simulink model "AcO_Ctrl_Geometric_headless_R2016a"  (R2016a)
settings: Solver=FixedStepDiscrete  StartTime=0.0  StopTime=simulation_duration  FixedStep=Ts  RelTol=1e-3
values from neighbouring files (symbols this model uses):
  M1_BeMo_d = zeros(7,M1_n_mode)    [AcO_Ctrl_headless_cfg.m]    (also in agws_cfg.m = 1e-6*bsxfun(@times,randn(7,M1_n_mode),scale); agws_fastTT_cfg.m = 1e-6*bsxfun(@times,randn(7,M1_n_mode),scale))
  M1_RiBo_d = zeros(7,6)    [AcO_Ctrl_headless_cfg.m]    (also in agws_cfg.m = [M1_Txyz0 M1_Rxyz0]; agws_fastTT_cfg.m = [M1_Txyz0 M1_Rxyz0])
  M2_RiBo_d = zeros(7,6)    [AcO_Ctrl_headless_cfg.m]    (also in agws_cfg.m = [M2_Txyz0 M2_Rxyz0]; agws_fastTT_cfg.m = [M2_Txyz0 M2_Rxyz0])
  Ts = 1/fs    (= 0.002)    [AcO_Ctrl_headless_cfg.m]    (also in agws_fastTT_cfg.m = 0.005)
undefined symbols (not defined in the file or in its folder): Az_C, CG2Hp, CG2Hp_S7, El_C, Fsmm, GIR_C, Hp2CG_f, Hp2CG_f_S7, HPdtf, HpK, KM2, M2_actdyn, M2_CG2Hp, M_LOS, MIMO_C, PTT2act, PTT2act_even, Q, sysd, TT2act, TT2act_even
undefined symbols (not defined in the file): on_axis_src_outputs
libraries: CEO x2
(part 5 of 6)

== system AcO_Ctrl_Geometric_headless_R2016a/Structural Dynamics V3.3/Structural Dynamics V3.3a/Structural Dynamics Plus CL Az El M1 force/M1 Sensing/senseM1S2 ==
  HP_D_cmd : Inport
  HP_D_face : Inport  Port=2
  HP_D_cell : Inport  Port=3
  Hp2CG_f : Gain  Gain=Hp2CG_f  Multiplication=Matrix(K*u)
  KHp : Gain  Gain=-HpK
  Sum1 : Sum  Inputs=-+|
  Sum9 : Sum  Inputs=-+|
  HardPoint_6DOF_Force : Outport
  wires:
  HP_D_face/1 -> Sum9/2
  HP_D_cmd/1 -> Sum1/1
  HP_D_cell/1 -> Sum9/1
  Hp2CG_f/1 -> HardPoint_6DOF_Force/1
  Sum9/1 -> Sum1/2
  Sum1/1 -> KHp/1
  KHp/1 -> Hp2CG_f/1

== system AcO_Ctrl_Geometric_headless_R2016a/Structural Dynamics V3.3/Structural Dynamics V3.3a/Structural Dynamics Plus CL Az El M1 force/M1 Sensing/senseM1S3 ==
  HP_D_cmd : Inport
  HP_D_face : Inport  Port=2
  HP_D_cell : Inport  Port=3
  Hp2CG_f : Gain  Gain=Hp2CG_f  Multiplication=Matrix(K*u)
  KHp : Gain  Gain=-HpK
  Sum1 : Sum  Inputs=-+|
  Sum9 : Sum  Inputs=-+|
  HardPoint_6DOF_Force : Outport
  wires:
  Hp2CG_f/1 -> HardPoint_6DOF_Force/1
  HP_D_cell/1 -> Sum9/1
  HP_D_cmd/1 -> Sum1/1
  HP_D_face/1 -> Sum9/2
  Sum9/1 -> Sum1/2
  Sum1/1 -> KHp/1
  KHp/1 -> Hp2CG_f/1

== system AcO_Ctrl_Geometric_headless_R2016a/Structural Dynamics V3.3/Structural Dynamics V3.3a/Structural Dynamics Plus CL Az El M1 force/M1 Sensing/senseM1S4 ==
  HP_D_cmd : Inport
  HP_D_face : Inport  Port=2
  HP_D_cell : Inport  Port=3
  Hp2CG_f : Gain  Gain=Hp2CG_f  Multiplication=Matrix(K*u)
  KHp : Gain  Gain=-HpK
  Sum1 : Sum  Inputs=-+|
  Sum9 : Sum  Inputs=-+|
  HardPoint_6DOF_Force : Outport
  wires:
  HP_D_face/1 -> Sum9/2
  HP_D_cmd/1 -> Sum1/1
  HP_D_cell/1 -> Sum9/1
  Hp2CG_f/1 -> HardPoint_6DOF_Force/1
  Sum9/1 -> Sum1/2
  Sum1/1 -> KHp/1
  KHp/1 -> Hp2CG_f/1

== system AcO_Ctrl_Geometric_headless_R2016a/Structural Dynamics V3.3/Structural Dynamics V3.3a/Structural Dynamics Plus CL Az El M1 force/M1 Sensing/senseM1S5 ==
  HP_D_cmd : Inport
  HP_D_face : Inport  Port=2
  HP_D_cell : Inport  Port=3
  Hp2CG_f : Gain  Gain=Hp2CG_f  Multiplication=Matrix(K*u)
  KHp : Gain  Gain=-HpK
  Sum1 : Sum  Inputs=-+|
  Sum9 : Sum  Inputs=-+|
  HardPoint_6DOF_Force : Outport
  wires:
  Hp2CG_f/1 -> HardPoint_6DOF_Force/1
  HP_D_cell/1 -> Sum9/1
  HP_D_cmd/1 -> Sum1/1
  HP_D_face/1 -> Sum9/2
  Sum9/1 -> Sum1/2
  Sum1/1 -> KHp/1
  KHp/1 -> Hp2CG_f/1

== system AcO_Ctrl_Geometric_headless_R2016a/Structural Dynamics V3.3/Structural Dynamics V3.3a/Structural Dynamics Plus CL Az El M1 force/M1 Sensing/senseM1S6 ==
  HP_D_cmd : Inport
  HP_D_face : Inport  Port=2
  HP_D_cell : Inport  Port=3
  Hp2CG_f : Gain  Gain=Hp2CG_f  Multiplication=Matrix(K*u)
  KHp : Gain  Gain=-HpK
  Sum1 : Sum  Inputs=-+|
  Sum9 : Sum  Inputs=-+|
  HardPoint_6DOF_Force : Outport
  wires:
  HP_D_face/1 -> Sum9/2
  HP_D_cmd/1 -> Sum1/1
  HP_D_cell/1 -> Sum9/1
  Hp2CG_f/1 -> HardPoint_6DOF_Force/1
  Sum9/1 -> Sum1/2
  Sum1/1 -> KHp/1
  KHp/1 -> Hp2CG_f/1

== system AcO_Ctrl_Geometric_headless_R2016a/Structural Dynamics V3.3/Structural Dynamics V3.3a/Structural Dynamics Plus CL Az El M1 force/M1 Sensing/senseM1S7 ==
  HP_D_cmd : Inport
  HP_D_face : Inport  Port=2
  HP_D_cell : Inport  Port=3
  Hp2CG_f_S7 : Gain  Gain=Hp2CG_f_S7  Multiplication=Matrix(K*u)
  KHp : Gain  Gain=-HpK
  Sum1 : Sum  Inputs=-+|
  Sum9 : Sum  Inputs=-+|
  HardPoint_6DOF_Force : Outport
  wires:
  Hp2CG_f_S7/1 -> HardPoint_6DOF_Force/1
  HP_D_cell/1 -> Sum9/1
  HP_D_cmd/1 -> Sum1/1
  HP_D_face/1 -> Sum9/2
  Sum9/1 -> Sum1/2
  Sum1/1 -> KHp/1
  KHp/1 -> Hp2CG_f_S7/1

== system AcO_Ctrl_Geometric_headless_R2016a/Structural Dynamics V3.3/Structural Dynamics V3.5.2/Structural Dynamics Plus CL Az El M1 force/M1 Force Control/ControlM1S1 ==
  In1 : Inport
  -1(2)3 : Gain  Gain=-1
  Actuator Model : DiscreteStateSpace  A=Q.A  B=Q.B  C=Q.C  D=Q.D  SampleTime=1/Fsmm
  MIMO Controller : Subsystem
  Out1 : Outport
  Out2 : Outport  Port=2
  wires:
  MIMO Controller/1(Out1) -> Actuator Model/1
  -1(2)3/1 -> Out2/1
  Actuator Model/1 -> -1(2)3/1, Out1/1
  In1/1 -> MIMO Controller/1(In1)

== system AcO_Ctrl_Geometric_headless_R2016a/Structural Dynamics V3.3/Structural Dynamics V3.5.2/Structural Dynamics Plus CL Az El M1 force/M1 Force Control/ControlM1S2 ==
  In1 : Inport
  -1(2)3 : Gain  Gain=-1
  Actuator Model : DiscreteStateSpace  A=Q.A  B=Q.B  C=Q.C  D=Q.D  SampleTime=1/Fsmm
  MIMO Controller : Subsystem
  Out1 : Outport
  Out2 : Outport  Port=2
  wires:
  In1/1 -> MIMO Controller/1(In1)
  Actuator Model/1 -> Out1/1, -1(2)3/1
  -1(2)3/1 -> Out2/1
  MIMO Controller/1(Out1) -> Actuator Model/1

== system AcO_Ctrl_Geometric_headless_R2016a/Structural Dynamics V3.3/Structural Dynamics V3.5.2/Structural Dynamics Plus CL Az El M1 force/M1 Force Control/ControlM1S3 ==
  In1 : Inport
  -1(2)3 : Gain  Gain=-1
  Actuator Model : DiscreteStateSpace  A=Q.A  B=Q.B  C=Q.C  D=Q.D  SampleTime=1/Fsmm
  MIMO Controller : Subsystem
  Out1 : Outport
  Out2 : Outport  Port=2
  wires:
  MIMO Controller/1(Out1) -> Actuator Model/1
  -1(2)3/1 -> Out2/1
  Actuator Model/1 -> -1(2)3/1, Out1/1
  In1/1 -> MIMO Controller/1(In1)

== system AcO_Ctrl_Geometric_headless_R2016a/Structural Dynamics V3.3/Structural Dynamics V3.5.2/Structural Dynamics Plus CL Az El M1 force/M1 Force Control/ControlM1S4 ==
  In1 : Inport
  -1(2)3 : Gain  Gain=-1
  Actuator Model : DiscreteStateSpace  A=Q.A  B=Q.B  C=Q.C  D=Q.D  SampleTime=1/Fsmm
  MIMO Controller : Subsystem
  Out1 : Outport
  Out2 : Outport  Port=2
  wires:
  In1/1 -> MIMO Controller/1(In1)
  Actuator Model/1 -> Out1/1, -1(2)3/1
  -1(2)3/1 -> Out2/1
  MIMO Controller/1(Out1) -> Actuator Model/1

== system AcO_Ctrl_Geometric_headless_R2016a/Structural Dynamics V3.3/Structural Dynamics V3.5.2/Structural Dynamics Plus CL Az El M1 force/M1 Force Control/ControlM1S5 ==
  In1 : Inport
  -1(2)3 : Gain  Gain=-1
  Actuator Model : DiscreteStateSpace  A=Q.A  B=Q.B  C=Q.C  D=Q.D  SampleTime=1/Fsmm
  MIMO Controller : Subsystem
  Out1 : Outport
  Out2 : Outport  Port=2
  wires:
  MIMO Controller/1(Out1) -> Actuator Model/1
  -1(2)3/1 -> Out2/1
  Actuator Model/1 -> -1(2)3/1, Out1/1
  In1/1 -> MIMO Controller/1(In1)

== system AcO_Ctrl_Geometric_headless_R2016a/Structural Dynamics V3.3/Structural Dynamics V3.5.2/Structural Dynamics Plus CL Az El M1 force/M1 Force Control/ControlM1S6 ==
  In1 : Inport
  -1(2)3 : Gain  Gain=-1
  Actuator Model : DiscreteStateSpace  A=Q.A  B=Q.B  C=Q.C  D=Q.D  SampleTime=1/Fsmm
  MIMO Controller : Subsystem
  Out1 : Outport
  Out2 : Outport  Port=2
  wires:
  In1/1 -> MIMO Controller/1(In1)
  Actuator Model/1 -> Out1/1, -1(2)3/1
  -1(2)3/1 -> Out2/1
  MIMO Controller/1(Out1) -> Actuator Model/1

== system AcO_Ctrl_Geometric_headless_R2016a/Structural Dynamics V3.3/Structural Dynamics V3.5.2/Structural Dynamics Plus CL Az El M1 force/M1 Force Control/ControlM1S7 ==
  In1 : Inport
  -1(2)3 : Gain  Gain=-1
  Actuator Model : DiscreteStateSpace  A=Q.A  B=Q.B  C=Q.C  D=Q.D  SampleTime=1/Fsmm
  MIMO Controller : Subsystem
  Out1 : Outport
  Out2 : Outport  Port=2
  wires:
  MIMO Controller/1(Out1) -> Actuator Model/1
  -1(2)3/1 -> Out2/1
  Actuator Model/1 -> -1(2)3/1, Out1/1
  In1/1 -> MIMO Controller/1(In1)

== system AcO_Ctrl_Geometric_headless_R2016a/Structural Dynamics V3.3/Structural Dynamics V3.5.2/Structural Dynamics Plus CL Az El M1 force/M1 Sensing/senseM1S1 ==
  HP_D_cmd : Inport
  HP_D_face : Inport  Port=2
  HP_D_cell : Inport  Port=3
  Hp2CG_f : Gain  Gain=Hp2CG_f  Multiplication=Matrix(K*u)
  KHp : Gain  Gain=-HpK
  Sum1 : Sum  Inputs=-+|
  Sum9 : Sum  Inputs=-+|
  HardPoint_6DOF_Force : Outport
  wires:
  Hp2CG_f/1 -> HardPoint_6DOF_Force/1
  HP_D_cell/1 -> Sum9/1
  HP_D_cmd/1 -> Sum1/1
  HP_D_face/1 -> Sum9/2
  Sum9/1 -> Sum1/2
  Sum1/1 -> KHp/1
  KHp/1 -> Hp2CG_f/1

== system AcO_Ctrl_Geometric_headless_R2016a/Structural Dynamics V3.3/Structural Dynamics V3.5.2/Structural Dynamics Plus CL Az El M1 force/M1 Sensing/senseM1S2 ==
  HP_D_cmd : Inport
  HP_D_face : Inport  Port=2
  HP_D_cell : Inport  Port=3
  Hp2CG_f : Gain  Gain=Hp2CG_f  Multiplication=Matrix(K*u)
  KHp : Gain  Gain=-HpK
  Scope : Scope
  Sum1 : Sum  Inputs=-+|
  Sum9 : Sum  Inputs=-+|
  HardPoint_6DOF_Force : Outport
  wires:
  HP_D_face/1 -> Sum9/2
  HP_D_cmd/1 -> Sum1/1
  Sum9/1 -> Scope/1, Sum1/2
  KHp/1 -> Hp2CG_f/1
  Hp2CG_f/1 -> HardPoint_6DOF_Force/1
  Sum1/1 -> KHp/1
  HP_D_cell/1 -> Sum9/1

== system AcO_Ctrl_Geometric_headless_R2016a/Structural Dynamics V3.3/Structural Dynamics V3.5.2/Structural Dynamics Plus CL Az El M1 force/M1 Sensing/senseM1S3 ==
  HP_D_cmd : Inport
  HP_D_face : Inport  Port=2
  HP_D_cell : Inport  Port=3
  Hp2CG_f : Gain  Gain=Hp2CG_f  Multiplication=Matrix(K*u)
  KHp : Gain  Gain=-HpK
  Sum1 : Sum  Inputs=-+|
  Sum9 : Sum  Inputs=-+|
  HardPoint_6DOF_Force : Outport
  wires:
  HP_D_face/1 -> Sum9/2
  HP_D_cmd/1 -> Sum1/1
  HP_D_cell/1 -> Sum9/1
  Hp2CG_f/1 -> HardPoint_6DOF_Force/1
  Sum9/1 -> Sum1/2
  Sum1/1 -> KHp/1
  KHp/1 -> Hp2CG_f/1

== system AcO_Ctrl_Geometric_headless_R2016a/Structural Dynamics V3.3/Structural Dynamics V3.5.2/Structural Dynamics Plus CL Az El M1 force/M1 Sensing/senseM1S4 ==
  HP_D_cmd : Inport
  HP_D_face : Inport  Port=2
  HP_D_cell : Inport  Port=3
  Hp2CG_f : Gain  Gain=Hp2CG_f  Multiplication=Matrix(K*u)
  KHp : Gain  Gain=-HpK
  Sum1 : Sum  Inputs=-+|
  Sum9 : Sum  Inputs=-+|
  HardPoint_6DOF_Force : Outport
  wires:
  Hp2CG_f/1 -> HardPoint_6DOF_Force/1
  HP_D_cell/1 -> Sum9/1
  HP_D_cmd/1 -> Sum1/1
  HP_D_face/1 -> Sum9/2
  Sum9/1 -> Sum1/2
  Sum1/1 -> KHp/1
  KHp/1 -> Hp2CG_f/1

== system AcO_Ctrl_Geometric_headless_R2016a/Structural Dynamics V3.3/Structural Dynamics V3.5.2/Structural Dynamics Plus CL Az El M1 force/M1 Sensing/senseM1S5 ==
  HP_D_cmd : Inport
  HP_D_face : Inport  Port=2
  HP_D_cell : Inport  Port=3
  Hp2CG_f : Gain  Gain=Hp2CG_f  Multiplication=Matrix(K*u)
  KHp : Gain  Gain=-HpK
  Sum1 : Sum  Inputs=-+|
  Sum9 : Sum  Inputs=-+|
  HardPoint_6DOF_Force : Outport
  wires:
  HP_D_face/1 -> Sum9/2
  HP_D_cmd/1 -> Sum1/1
  HP_D_cell/1 -> Sum9/1
  Hp2CG_f/1 -> HardPoint_6DOF_Force/1
  Sum9/1 -> Sum1/2
  Sum1/1 -> KHp/1
  KHp/1 -> Hp2CG_f/1

== system AcO_Ctrl_Geometric_headless_R2016a/Structural Dynamics V3.3/Structural Dynamics V3.5.2/Structural Dynamics Plus CL Az El M1 force/M1 Sensing/senseM1S6 ==
  HP_D_cmd : Inport
  HP_D_face : Inport  Port=2
  HP_D_cell : Inport  Port=3
  Hp2CG_f : Gain  Gain=Hp2CG_f  Multiplication=Matrix(K*u)
  KHp : Gain  Gain=-HpK
  Sum1 : Sum  Inputs=-+|
  Sum9 : Sum  Inputs=-+|
  HardPoint_6DOF_Force : Outport
  wires:
  Hp2CG_f/1 -> HardPoint_6DOF_Force/1
  HP_D_cell/1 -> Sum9/1
  HP_D_cmd/1 -> Sum1/1
  HP_D_face/1 -> Sum9/2
  Sum9/1 -> Sum1/2
  Sum1/1 -> KHp/1
  KHp/1 -> Hp2CG_f/1

== system AcO_Ctrl_Geometric_headless_R2016a/Structural Dynamics V3.3/Structural Dynamics V3.5.2/Structural Dynamics Plus CL Az El M1 force/M1 Sensing/senseM1S7 ==
  HP_D_cmd : Inport
  HP_D_face : Inport  Port=2
  HP_D_cell : Inport  Port=3
  Hp2CG_f_S7 : Gain  Gain=Hp2CG_f_S7  Multiplication=Matrix(K*u)
  KHp : Gain  Gain=-HpK
  Sum1 : Sum  Inputs=-+|
  Sum9 : Sum  Inputs=-+|
  HardPoint_6DOF_Force : Outport
  wires:
  HP_D_face/1 -> Sum9/2
  HP_D_cmd/1 -> Sum1/1
  HP_D_cell/1 -> Sum9/1
  Hp2CG_f_S7/1 -> HardPoint_6DOF_Force/1
  Sum9/1 -> Sum1/2
  Sum1/1 -> KHp/1
  KHp/1 -> Hp2CG_f_S7/1

== system AcO_Ctrl_Geometric_headless_R2016a/Structural Dynamics V3.3/Structural Dynamics V3.5.3/Structural Dynamics Plus CL Az El M1 force/M1 Force Control/ControlM1S1 ==
  In1 : Inport
  -1(2)3 : Gain  Gain=-1
  Actuator Model : DiscreteStateSpace  A=Q.A  B=Q.B  C=Q.C  D=Q.D  SampleTime=1/Fsmm
  MIMO Controller : Subsystem
  Out1 : Outport
  Out2 : Outport  Port=2
  wires:
  MIMO Controller/1(Out1) -> Actuator Model/1
  -1(2)3/1 -> Out2/1
  Actuator Model/1 -> -1(2)3/1, Out1/1
  In1/1 -> MIMO Controller/1(In1)

== system AcO_Ctrl_Geometric_headless_R2016a/Structural Dynamics V3.3/Structural Dynamics V3.5.3/Structural Dynamics Plus CL Az El M1 force/M1 Force Control/ControlM1S2 ==
  In1 : Inport
  -1(2)3 : Gain  Gain=-1
  Actuator Model : DiscreteStateSpace  A=Q.A  B=Q.B  C=Q.C  D=Q.D  SampleTime=1/Fsmm
  MIMO Controller : Subsystem
  Out1 : Outport
  Out2 : Outport  Port=2
  wires:
  In1/1 -> MIMO Controller/1(In1)
  Actuator Model/1 -> Out1/1, -1(2)3/1
  -1(2)3/1 -> Out2/1
  MIMO Controller/1(Out1) -> Actuator Model/1

== system AcO_Ctrl_Geometric_headless_R2016a/Structural Dynamics V3.3/Structural Dynamics V3.5.3/Structural Dynamics Plus CL Az El M1 force/M1 Force Control/ControlM1S3 ==
  In1 : Inport
  -1(2)3 : Gain  Gain=-1
  Actuator Model : DiscreteStateSpace  A=Q.A  B=Q.B  C=Q.C  D=Q.D  SampleTime=1/Fsmm
  MIMO Controller : Subsystem
  Out1 : Outport
  Out2 : Outport  Port=2
  wires:
  MIMO Controller/1(Out1) -> Actuator Model/1
  -1(2)3/1 -> Out2/1
  Actuator Model/1 -> -1(2)3/1, Out1/1
  In1/1 -> MIMO Controller/1(In1)

== system AcO_Ctrl_Geometric_headless_R2016a/Structural Dynamics V3.3/Structural Dynamics V3.5.3/Structural Dynamics Plus CL Az El M1 force/M1 Force Control/ControlM1S4 ==
  In1 : Inport
  -1(2)3 : Gain  Gain=-1
  Actuator Model : DiscreteStateSpace  A=Q.A  B=Q.B  C=Q.C  D=Q.D  SampleTime=1/Fsmm
  MIMO Controller : Subsystem
  Out1 : Outport
  Out2 : Outport  Port=2
  wires:
  In1/1 -> MIMO Controller/1(In1)
  Actuator Model/1 -> Out1/1, -1(2)3/1
  -1(2)3/1 -> Out2/1
  MIMO Controller/1(Out1) -> Actuator Model/1

== system AcO_Ctrl_Geometric_headless_R2016a/Structural Dynamics V3.3/Structural Dynamics V3.5.3/Structural Dynamics Plus CL Az El M1 force/M1 Force Control/ControlM1S5 ==
  In1 : Inport
  -1(2)3 : Gain  Gain=-1
  Actuator Model : DiscreteStateSpace  A=Q.A  B=Q.B  C=Q.C  D=Q.D  SampleTime=1/Fsmm
  MIMO Controller : Subsystem
  Out1 : Outport
  Out2 : Outport  Port=2
  wires:
  MIMO Controller/1(Out1) -> Actuator Model/1
  -1(2)3/1 -> Out2/1
  Actuator Model/1 -> -1(2)3/1, Out1/1
  In1/1 -> MIMO Controller/1(In1)

== system AcO_Ctrl_Geometric_headless_R2016a/Structural Dynamics V3.3/Structural Dynamics V3.5.3/Structural Dynamics Plus CL Az El M1 force/M1 Force Control/ControlM1S6 ==
  In1 : Inport
  -1(2)3 : Gain  Gain=-1
  Actuator Model : DiscreteStateSpace  A=Q.A  B=Q.B  C=Q.C  D=Q.D  SampleTime=1/Fsmm
  MIMO Controller : Subsystem
  Out1 : Outport
  Out2 : Outport  Port=2
  wires:
  In1/1 -> MIMO Controller/1(In1)
  Actuator Model/1 -> Out1/1, -1(2)3/1
  -1(2)3/1 -> Out2/1
  MIMO Controller/1(Out1) -> Actuator Model/1

== system AcO_Ctrl_Geometric_headless_R2016a/Structural Dynamics V3.3/Structural Dynamics V3.5.3/Structural Dynamics Plus CL Az El M1 force/M1 Force Control/ControlM1S7 ==
  In1 : Inport
  -1(2)3 : Gain  Gain=-1
  Actuator Model : DiscreteStateSpace  A=Q.A  B=Q.B  C=Q.C  D=Q.D  SampleTime=1/Fsmm
  MIMO Controller : Subsystem
  Out1 : Outport
  Out2 : Outport  Port=2
  wires:
  MIMO Controller/1(Out1) -> Actuator Model/1
  -1(2)3/1 -> Out2/1
  Actuator Model/1 -> -1(2)3/1, Out1/1
  In1/1 -> MIMO Controller/1(In1)

== system AcO_Ctrl_Geometric_headless_R2016a/Structural Dynamics V3.3/Structural Dynamics V3.5.3/Structural Dynamics Plus CL Az El M1 force/M1 Sensing/senseM1S1 ==
  HP_D_cmd : Inport
  HP_D_face : Inport  Port=2
  HP_D_cell : Inport  Port=3
  Hp2CG_f : Gain  Gain=Hp2CG_f  Multiplication=Matrix(K*u)
  KHp : Gain  Gain=-HpK
  Sum1 : Sum  Inputs=-+|
  Sum9 : Sum  Inputs=-+|
  HardPoint_6DOF_Force : Outport
  wires:
  Hp2CG_f/1 -> HardPoint_6DOF_Force/1
  HP_D_cell/1 -> Sum9/1
  HP_D_cmd/1 -> Sum1/1
  HP_D_face/1 -> Sum9/2
  Sum9/1 -> Sum1/2
  Sum1/1 -> KHp/1
  KHp/1 -> Hp2CG_f/1

== system AcO_Ctrl_Geometric_headless_R2016a/Structural Dynamics V3.3/Structural Dynamics V3.5.3/Structural Dynamics Plus CL Az El M1 force/M1 Sensing/senseM1S2 ==
  HP_D_cmd : Inport
  HP_D_face : Inport  Port=2
  HP_D_cell : Inport  Port=3
  Hp2CG_f : Gain  Gain=Hp2CG_f  Multiplication=Matrix(K*u)
  KHp : Gain  Gain=-HpK
  Scope : Scope
  Sum1 : Sum  Inputs=-+|
  Sum9 : Sum  Inputs=-+|
  HardPoint_6DOF_Force : Outport
  wires:
  HP_D_face/1 -> Sum9/2
  HP_D_cmd/1 -> Sum1/1
  Sum9/1 -> Scope/1, Sum1/2
  KHp/1 -> Hp2CG_f/1
  Hp2CG_f/1 -> HardPoint_6DOF_Force/1
  Sum1/1 -> KHp/1
  HP_D_cell/1 -> Sum9/1

== system AcO_Ctrl_Geometric_headless_R2016a/Structural Dynamics V3.3/Structural Dynamics V3.5.3/Structural Dynamics Plus CL Az El M1 force/M1 Sensing/senseM1S3 ==
  HP_D_cmd : Inport
  HP_D_face : Inport  Port=2
  HP_D_cell : Inport  Port=3
  Hp2CG_f : Gain  Gain=Hp2CG_f  Multiplication=Matrix(K*u)
  KHp : Gain  Gain=-HpK
  Sum1 : Sum  Inputs=-+|
  Sum9 : Sum  Inputs=-+|
  HardPoint_6DOF_Force : Outport
  wires:
  HP_D_face/1 -> Sum9/2
  HP_D_cmd/1 -> Sum1/1
  HP_D_cell/1 -> Sum9/1
  Hp2CG_f/1 -> HardPoint_6DOF_Force/1
  Sum9/1 -> Sum1/2
  Sum1/1 -> KHp/1
  KHp/1 -> Hp2CG_f/1

== system AcO_Ctrl_Geometric_headless_R2016a/Structural Dynamics V3.3/Structural Dynamics V3.5.3/Structural Dynamics Plus CL Az El M1 force/M1 Sensing/senseM1S4 ==
  HP_D_cmd : Inport
  HP_D_face : Inport  Port=2
  HP_D_cell : Inport  Port=3
  Hp2CG_f : Gain  Gain=Hp2CG_f  Multiplication=Matrix(K*u)
  KHp : Gain  Gain=-HpK
  Sum1 : Sum  Inputs=-+|
  Sum9 : Sum  Inputs=-+|
  HardPoint_6DOF_Force : Outport
  wires:
  Hp2CG_f/1 -> HardPoint_6DOF_Force/1
  HP_D_cell/1 -> Sum9/1
  HP_D_cmd/1 -> Sum1/1
  HP_D_face/1 -> Sum9/2
  Sum9/1 -> Sum1/2
  Sum1/1 -> KHp/1
  KHp/1 -> Hp2CG_f/1

== system AcO_Ctrl_Geometric_headless_R2016a/Structural Dynamics V3.3/Structural Dynamics V3.5.3/Structural Dynamics Plus CL Az El M1 force/M1 Sensing/senseM1S5 ==
  HP_D_cmd : Inport
  HP_D_face : Inport  Port=2
  HP_D_cell : Inport  Port=3
  Hp2CG_f : Gain  Gain=Hp2CG_f  Multiplication=Matrix(K*u)
  KHp : Gain  Gain=-HpK
  Sum1 : Sum  Inputs=-+|
  Sum9 : Sum  Inputs=-+|
  HardPoint_6DOF_Force : Outport
  wires:
  HP_D_face/1 -> Sum9/2
  HP_D_cmd/1 -> Sum1/1
  HP_D_cell/1 -> Sum9/1
  Hp2CG_f/1 -> HardPoint_6DOF_Force/1
  Sum9/1 -> Sum1/2
  Sum1/1 -> KHp/1
  KHp/1 -> Hp2CG_f/1

== system AcO_Ctrl_Geometric_headless_R2016a/Structural Dynamics V3.3/Structural Dynamics V3.5.3/Structural Dynamics Plus CL Az El M1 force/M1 Sensing/senseM1S6 ==
  HP_D_cmd : Inport
  HP_D_face : Inport  Port=2
  HP_D_cell : Inport  Port=3
  Hp2CG_f : Gain  Gain=Hp2CG_f  Multiplication=Matrix(K*u)
  KHp : Gain  Gain=-HpK
  Sum1 : Sum  Inputs=-+|
  Sum9 : Sum  Inputs=-+|
  HardPoint_6DOF_Force : Outport
  wires:
  Hp2CG_f/1 -> HardPoint_6DOF_Force/1
  HP_D_cell/1 -> Sum9/1
  HP_D_cmd/1 -> Sum1/1
  HP_D_face/1 -> Sum9/2
  Sum9/1 -> Sum1/2
  Sum1/1 -> KHp/1
  KHp/1 -> Hp2CG_f/1

== system AcO_Ctrl_Geometric_headless_R2016a/Structural Dynamics V3.3/Structural Dynamics V3.5.3/Structural Dynamics Plus CL Az El M1 force/M1 Sensing/senseM1S7 ==
  HP_D_cmd : Inport
  HP_D_face : Inport  Port=2
  HP_D_cell : Inport  Port=3
  Hp2CG_f_S7 : Gain  Gain=Hp2CG_f_S7  Multiplication=Matrix(K*u)
  KHp : Gain  Gain=-HpK
  Sum1 : Sum  Inputs=-+|
  Sum9 : Sum  Inputs=-+|
  HardPoint_6DOF_Force : Outport
  wires:
  HP_D_face/1 -> Sum9/2
  HP_D_cmd/1 -> Sum1/1
  HP_D_cell/1 -> Sum9/1
  Hp2CG_f_S7/1 -> HardPoint_6DOF_Force/1
  Sum9/1 -> Sum1/2
  Sum1/1 -> KHp/1
  KHp/1 -> Hp2CG_f_S7/1

== system AcO_Ctrl_Geometric_headless_R2016a/Structural Dynamics V3.3/Structural Dynamics V3.3/Structural Dynamics Plus CL Az El M1 force/M1 Force Control/ControlM1S1/MIMO Controller ==
  In1 : Inport
  Demux1 : Demux  Outputs=6
  Gain{,1..5} (6 alike) : Gain
  Mux1 : Mux  Inputs=6
  R1 Controller : DiscreteTransferFcn  Numerator=MIMO_C(4,4).num{1}  Denominator=MIMO_C(4,4).den{1}
  R2 Controller : DiscreteTransferFcn  Numerator=MIMO_C(5,5).num{1}  Denominator=MIMO_C(5,5).den{1}
  R3 Controller : DiscreteTransferFcn  Numerator=MIMO_C(6,6).num{1}  Denominator=MIMO_C(6,6).den{1}
  T1 Controller : DiscreteTransferFcn  Numerator=MIMO_C(1,1).num{1}  Denominator=MIMO_C(1,1).den{1}
  T2 Controller : DiscreteTransferFcn  Numerator=MIMO_C(2,2).num{1}  Denominator=MIMO_C(2,2).den{1}
  T3 Controller : DiscreteTransferFcn  Numerator=MIMO_C(3,3).num{1}  Denominator=MIMO_C(3,3).den{1}
  Out1 : Outport
  wires:
  Gain5/1 -> T3 Controller/1
  Gain4/1 -> R3 Controller/1
  Gain3/1 -> R2 Controller/1
  Gain2/1 -> R1 Controller/1
  Gain1/1 -> T2 Controller/1
  Gain/1 -> T1 Controller/1
  Mux1/1 -> Out1/1
  T1 Controller/1 -> Mux1/1
  T2 Controller/1 -> Mux1/2
  T3 Controller/1 -> Mux1/3
  R1 Controller/1 -> Mux1/4
  R2 Controller/1 -> Mux1/5
  R3 Controller/1 -> Mux1/6
  Demux1/6 -> Gain4/1
  Demux1/5 -> Gain3/1
  Demux1/4 -> Gain2/1
  Demux1/3 -> Gain5/1
  Demux1/2 -> Gain1/1
  Demux1/1 -> Gain/1
  In1/1 -> Demux1/1

== system AcO_Ctrl_Geometric_headless_R2016a/Structural Dynamics V3.3/Structural Dynamics V3.3/Structural Dynamics Plus CL Az El M1 force/M1 Force Control/ControlM1S2/MIMO Controller ==
  In1 : Inport
  Demux1 : Demux  Outputs=6
  Gain{,1..5} (6 alike) : Gain
  Mux1 : Mux  Inputs=6
  R1 Controller : DiscreteTransferFcn  Numerator=MIMO_C(4,4).num{1}  Denominator=MIMO_C(4,4).den{1}
  R2 Controller : DiscreteTransferFcn  Numerator=MIMO_C(5,5).num{1}  Denominator=MIMO_C(5,5).den{1}
  R3 Controller : DiscreteTransferFcn  Numerator=MIMO_C(6,6).num{1}  Denominator=MIMO_C(6,6).den{1}
  T1 Controller : DiscreteTransferFcn  Numerator=MIMO_C(1,1).num{1}  Denominator=MIMO_C(1,1).den{1}
  T2 Controller : DiscreteTransferFcn  Numerator=MIMO_C(2,2).num{1}  Denominator=MIMO_C(2,2).den{1}
  T3 Controller : DiscreteTransferFcn  Numerator=MIMO_C(3,3).num{1}  Denominator=MIMO_C(3,3).den{1}
  Out1 : Outport
  wires:
  In1/1 -> Demux1/1
  Demux1/1 -> Gain/1
  Demux1/2 -> Gain1/1
  Demux1/3 -> Gain5/1
  Demux1/4 -> Gain2/1
  Demux1/5 -> Gain3/1
  Demux1/6 -> Gain4/1
  R3 Controller/1 -> Mux1/6
  R2 Controller/1 -> Mux1/5
  R1 Controller/1 -> Mux1/4
  T3 Controller/1 -> Mux1/3
  T2 Controller/1 -> Mux1/2
  T1 Controller/1 -> Mux1/1
  Mux1/1 -> Out1/1
  Gain/1 -> T1 Controller/1
  Gain1/1 -> T2 Controller/1
  Gain2/1 -> R1 Controller/1
  Gain3/1 -> R2 Controller/1
  Gain4/1 -> R3 Controller/1
  Gain5/1 -> T3 Controller/1

== system AcO_Ctrl_Geometric_headless_R2016a/Structural Dynamics V3.3/Structural Dynamics V3.3/Structural Dynamics Plus CL Az El M1 force/M1 Force Control/ControlM1S3/MIMO Controller ==
  In1 : Inport
  Demux1 : Demux  Outputs=6
  Gain{,1..5} (6 alike) : Gain
  Mux1 : Mux  Inputs=6
  R1 Controller : DiscreteTransferFcn  Numerator=MIMO_C(4,4).num{1}  Denominator=MIMO_C(4,4).den{1}
  R2 Controller : DiscreteTransferFcn  Numerator=MIMO_C(5,5).num{1}  Denominator=MIMO_C(5,5).den{1}
  R3 Controller : DiscreteTransferFcn  Numerator=MIMO_C(6,6).num{1}  Denominator=MIMO_C(6,6).den{1}
  T1 Controller : DiscreteTransferFcn  Numerator=MIMO_C(1,1).num{1}  Denominator=MIMO_C(1,1).den{1}
  T2 Controller : DiscreteTransferFcn  Numerator=MIMO_C(2,2).num{1}  Denominator=MIMO_C(2,2).den{1}
  T3 Controller : DiscreteTransferFcn  Numerator=MIMO_C(3,3).num{1}  Denominator=MIMO_C(3,3).den{1}
  Out1 : Outport
  wires:
  Gain5/1 -> T3 Controller/1
  Gain4/1 -> R3 Controller/1
  Gain3/1 -> R2 Controller/1
  Gain2/1 -> R1 Controller/1
  Gain1/1 -> T2 Controller/1
  Gain/1 -> T1 Controller/1
  Mux1/1 -> Out1/1
  T1 Controller/1 -> Mux1/1
  T2 Controller/1 -> Mux1/2
  T3 Controller/1 -> Mux1/3
  R1 Controller/1 -> Mux1/4
  R2 Controller/1 -> Mux1/5
  R3 Controller/1 -> Mux1/6
  Demux1/6 -> Gain4/1
  Demux1/5 -> Gain3/1
  Demux1/4 -> Gain2/1
  Demux1/3 -> Gain5/1
  Demux1/2 -> Gain1/1
  Demux1/1 -> Gain/1
  In1/1 -> Demux1/1

== system AcO_Ctrl_Geometric_headless_R2016a/Structural Dynamics V3.3/Structural Dynamics V3.3/Structural Dynamics Plus CL Az El M1 force/M1 Force Control/ControlM1S4/MIMO Controller ==
  In1 : Inport
  Demux1 : Demux  Outputs=6
  Gain{,1..5} (6 alike) : Gain
  Mux1 : Mux  Inputs=6
  R1 Controller : DiscreteTransferFcn  Numerator=MIMO_C(4,4).num{1}  Denominator=MIMO_C(4,4).den{1}
  R2 Controller : DiscreteTransferFcn  Numerator=MIMO_C(5,5).num{1}  Denominator=MIMO_C(5,5).den{1}
  R3 Controller : DiscreteTransferFcn  Numerator=MIMO_C(6,6).num{1}  Denominator=MIMO_C(6,6).den{1}
  T1 Controller : DiscreteTransferFcn  Numerator=MIMO_C(1,1).num{1}  Denominator=MIMO_C(1,1).den{1}
  T2 Controller : DiscreteTransferFcn  Numerator=MIMO_C(2,2).num{1}  Denominator=MIMO_C(2,2).den{1}
  T3 Controller : DiscreteTransferFcn  Numerator=MIMO_C(3,3).num{1}  Denominator=MIMO_C(3,3).den{1}
  Out1 : Outport
  wires:
  In1/1 -> Demux1/1
  Demux1/1 -> Gain/1
  Demux1/2 -> Gain1/1
  Demux1/3 -> Gain5/1
  Demux1/4 -> Gain2/1
  Demux1/5 -> Gain3/1
  Demux1/6 -> Gain4/1
  R3 Controller/1 -> Mux1/6
  R2 Controller/1 -> Mux1/5
  R1 Controller/1 -> Mux1/4
  T3 Controller/1 -> Mux1/3
  T2 Controller/1 -> Mux1/2
  T1 Controller/1 -> Mux1/1
  Mux1/1 -> Out1/1
  Gain/1 -> T1 Controller/1
  Gain1/1 -> T2 Controller/1
  Gain2/1 -> R1 Controller/1
  Gain3/1 -> R2 Controller/1
  Gain4/1 -> R3 Controller/1
  Gain5/1 -> T3 Controller/1

== system AcO_Ctrl_Geometric_headless_R2016a/Structural Dynamics V3.3/Structural Dynamics V3.3/Structural Dynamics Plus CL Az El M1 force/M1 Force Control/ControlM1S5/MIMO Controller ==
  In1 : Inport
  Demux1 : Demux  Outputs=6
  Gain{,1..5} (6 alike) : Gain
  Mux1 : Mux  Inputs=6
  R1 Controller : DiscreteTransferFcn  Numerator=MIMO_C(4,4).num{1}  Denominator=MIMO_C(4,4).den{1}
  R2 Controller : DiscreteTransferFcn  Numerator=MIMO_C(5,5).num{1}  Denominator=MIMO_C(5,5).den{1}
  R3 Controller : DiscreteTransferFcn  Numerator=MIMO_C(6,6).num{1}  Denominator=MIMO_C(6,6).den{1}
  T1 Controller : DiscreteTransferFcn  Numerator=MIMO_C(1,1).num{1}  Denominator=MIMO_C(1,1).den{1}
  T2 Controller : DiscreteTransferFcn  Numerator=MIMO_C(2,2).num{1}  Denominator=MIMO_C(2,2).den{1}
  T3 Controller : DiscreteTransferFcn  Numerator=MIMO_C(3,3).num{1}  Denominator=MIMO_C(3,3).den{1}
  Out1 : Outport
  wires:
  Gain5/1 -> T3 Controller/1
  Gain4/1 -> R3 Controller/1
  Gain3/1 -> R2 Controller/1
  Gain2/1 -> R1 Controller/1
  Gain1/1 -> T2 Controller/1
  Gain/1 -> T1 Controller/1
  Mux1/1 -> Out1/1
  T1 Controller/1 -> Mux1/1
  T2 Controller/1 -> Mux1/2
  T3 Controller/1 -> Mux1/3
  R1 Controller/1 -> Mux1/4
  R2 Controller/1 -> Mux1/5
  R3 Controller/1 -> Mux1/6
  Demux1/6 -> Gain4/1
  Demux1/5 -> Gain3/1
  Demux1/4 -> Gain2/1
  Demux1/3 -> Gain5/1
  Demux1/2 -> Gain1/1
  Demux1/1 -> Gain/1
  In1/1 -> Demux1/1

== system AcO_Ctrl_Geometric_headless_R2016a/Structural Dynamics V3.3/Structural Dynamics V3.3/Structural Dynamics Plus CL Az El M1 force/M1 Force Control/ControlM1S6/MIMO Controller ==
  In1 : Inport
  Demux1 : Demux  Outputs=6
  Gain{,1..5} (6 alike) : Gain
  Mux1 : Mux  Inputs=6
  R1 Controller : DiscreteTransferFcn  Numerator=MIMO_C(4,4).num{1}  Denominator=MIMO_C(4,4).den{1}
  R2 Controller : DiscreteTransferFcn  Numerator=MIMO_C(5,5).num{1}  Denominator=MIMO_C(5,5).den{1}
  R3 Controller : DiscreteTransferFcn  Numerator=MIMO_C(6,6).num{1}  Denominator=MIMO_C(6,6).den{1}
  T1 Controller : DiscreteTransferFcn  Numerator=MIMO_C(1,1).num{1}  Denominator=MIMO_C(1,1).den{1}
  T2 Controller : DiscreteTransferFcn  Numerator=MIMO_C(2,2).num{1}  Denominator=MIMO_C(2,2).den{1}
  T3 Controller : DiscreteTransferFcn  Numerator=MIMO_C(3,3).num{1}  Denominator=MIMO_C(3,3).den{1}
  Out1 : Outport
  wires:
  In1/1 -> Demux1/1
  Demux1/1 -> Gain/1
  Demux1/2 -> Gain1/1
  Demux1/3 -> Gain5/1
  Demux1/4 -> Gain2/1
  Demux1/5 -> Gain3/1
  Demux1/6 -> Gain4/1
  R3 Controller/1 -> Mux1/6
  R2 Controller/1 -> Mux1/5
  R1 Controller/1 -> Mux1/4
  T3 Controller/1 -> Mux1/3
  T2 Controller/1 -> Mux1/2
  T1 Controller/1 -> Mux1/1
  Mux1/1 -> Out1/1
  Gain/1 -> T1 Controller/1
  Gain1/1 -> T2 Controller/1
  Gain2/1 -> R1 Controller/1
  Gain3/1 -> R2 Controller/1
  Gain4/1 -> R3 Controller/1
  Gain5/1 -> T3 Controller/1

== system AcO_Ctrl_Geometric_headless_R2016a/Structural Dynamics V3.3/Structural Dynamics V3.3/Structural Dynamics Plus CL Az El M1 force/M1 Force Control/ControlM1S7/MIMO Controller ==
  In1 : Inport
  Demux1 : Demux  Outputs=6
  Gain{,1..5} (6 alike) : Gain
  Mux1 : Mux  Inputs=6
  R1 Controller : DiscreteTransferFcn  Numerator=MIMO_C(4,4).num{1}  Denominator=MIMO_C(4,4).den{1}
  R2 Controller : DiscreteTransferFcn  Numerator=MIMO_C(5,5).num{1}  Denominator=MIMO_C(5,5).den{1}
  R3 Controller : DiscreteTransferFcn  Numerator=MIMO_C(6,6).num{1}  Denominator=MIMO_C(6,6).den{1}
  T1 Controller : DiscreteTransferFcn  Numerator=MIMO_C(1,1).num{1}  Denominator=MIMO_C(1,1).den{1}
  T2 Controller : DiscreteTransferFcn  Numerator=MIMO_C(2,2).num{1}  Denominator=MIMO_C(2,2).den{1}
  T3 Controller : DiscreteTransferFcn  Numerator=MIMO_C(3,3).num{1}  Denominator=MIMO_C(3,3).den{1}
  Out1 : Outport
  wires:
  In1/1 -> Demux1/1
  Demux1/1 -> Gain/1
  Demux1/2 -> Gain1/1
  Demux1/3 -> Gain5/1
  Demux1/4 -> Gain2/1
  Demux1/5 -> Gain3/1
  Demux1/6 -> Gain4/1
  R3 Controller/1 -> Mux1/6
  R2 Controller/1 -> Mux1/5
  R1 Controller/1 -> Mux1/4
  T3 Controller/1 -> Mux1/3
  T2 Controller/1 -> Mux1/2
  T1 Controller/1 -> Mux1/1
  Mux1/1 -> Out1/1
  Gain/1 -> T1 Controller/1
  Gain1/1 -> T2 Controller/1
  Gain2/1 -> R1 Controller/1
  Gain3/1 -> R2 Controller/1
  Gain4/1 -> R3 Controller/1
  Gain5/1 -> T3 Controller/1

== system AcO_Ctrl_Geometric_headless_R2016a/Structural Dynamics V3.3/Structural Dynamics V3.3a/Structural Dynamics Plus CL Az El M1 force/M1 Force Control/ControlM1S1/MIMO Controller ==
  In1 : Inport
  Demux1 : Demux  Outputs=6
  Gain{,1..5} (6 alike) : Gain
  Mux1 : Mux  Inputs=6
  R1 Controller : DiscreteTransferFcn  Numerator=MIMO_C(4,4).num{1}  Denominator=MIMO_C(4,4).den{1}
  R2 Controller : DiscreteTransferFcn  Numerator=MIMO_C(5,5).num{1}  Denominator=MIMO_C(5,5).den{1}
  R3 Controller : DiscreteTransferFcn  Numerator=MIMO_C(6,6).num{1}  Denominator=MIMO_C(6,6).den{1}
  T1 Controller : DiscreteTransferFcn  Numerator=MIMO_C(1,1).num{1}  Denominator=MIMO_C(1,1).den{1}
  T2 Controller : DiscreteTransferFcn  Numerator=MIMO_C(2,2).num{1}  Denominator=MIMO_C(2,2).den{1}
  T3 Controller : DiscreteTransferFcn  Numerator=MIMO_C(3,3).num{1}  Denominator=MIMO_C(3,3).den{1}
  Out1 : Outport
  wires:
  In1/1 -> Demux1/1
  Demux1/1 -> Gain/1
  Demux1/2 -> Gain1/1
  Demux1/3 -> Gain5/1
  Demux1/4 -> Gain2/1
  Demux1/5 -> Gain3/1
  Demux1/6 -> Gain4/1
  R3 Controller/1 -> Mux1/6
  R2 Controller/1 -> Mux1/5
  R1 Controller/1 -> Mux1/4
  T3 Controller/1 -> Mux1/3
  T2 Controller/1 -> Mux1/2
  T1 Controller/1 -> Mux1/1
  Mux1/1 -> Out1/1
  Gain/1 -> T1 Controller/1
  Gain1/1 -> T2 Controller/1
  Gain2/1 -> R1 Controller/1
  Gain3/1 -> R2 Controller/1
  Gain4/1 -> R3 Controller/1
  Gain5/1 -> T3 Controller/1

== system AcO_Ctrl_Geometric_headless_R2016a/Structural Dynamics V3.3/Structural Dynamics V3.3a/Structural Dynamics Plus CL Az El M1 force/M1 Force Control/ControlM1S2/MIMO Controller ==
  In1 : Inport
  Demux1 : Demux  Outputs=6
  Gain{,1..5} (6 alike) : Gain
  Mux1 : Mux  Inputs=6
  R1 Controller : DiscreteTransferFcn  Numerator=MIMO_C(4,4).num{1}  Denominator=MIMO_C(4,4).den{1}
  R2 Controller : DiscreteTransferFcn  Numerator=MIMO_C(5,5).num{1}  Denominator=MIMO_C(5,5).den{1}
  R3 Controller : DiscreteTransferFcn  Numerator=MIMO_C(6,6).num{1}  Denominator=MIMO_C(6,6).den{1}
  T1 Controller : DiscreteTransferFcn  Numerator=MIMO_C(1,1).num{1}  Denominator=MIMO_C(1,1).den{1}
  T2 Controller : DiscreteTransferFcn  Numerator=MIMO_C(2,2).num{1}  Denominator=MIMO_C(2,2).den{1}
  T3 Controller : DiscreteTransferFcn  Numerator=MIMO_C(3,3).num{1}  Denominator=MIMO_C(3,3).den{1}
  Out1 : Outport
  wires:
  Gain5/1 -> T3 Controller/1
  Gain4/1 -> R3 Controller/1
  Gain3/1 -> R2 Controller/1
  Gain2/1 -> R1 Controller/1
  Gain1/1 -> T2 Controller/1
  Gain/1 -> T1 Controller/1
  Mux1/1 -> Out1/1
  T1 Controller/1 -> Mux1/1
  T2 Controller/1 -> Mux1/2
  T3 Controller/1 -> Mux1/3
  R1 Controller/1 -> Mux1/4
  R2 Controller/1 -> Mux1/5
  R3 Controller/1 -> Mux1/6
  Demux1/6 -> Gain4/1
  Demux1/5 -> Gain3/1
  Demux1/4 -> Gain2/1
  Demux1/3 -> Gain5/1
  Demux1/2 -> Gain1/1
  Demux1/1 -> Gain/1
  In1/1 -> Demux1/1

== system AcO_Ctrl_Geometric_headless_R2016a/Structural Dynamics V3.3/Structural Dynamics V3.3a/Structural Dynamics Plus CL Az El M1 force/M1 Force Control/ControlM1S3/MIMO Controller ==
  In1 : Inport
  Demux1 : Demux  Outputs=6
  Gain{,1..5} (6 alike) : Gain
  Mux1 : Mux  Inputs=6
  R1 Controller : DiscreteTransferFcn  Numerator=MIMO_C(4,4).num{1}  Denominator=MIMO_C(4,4).den{1}
  R2 Controller : DiscreteTransferFcn  Numerator=MIMO_C(5,5).num{1}  Denominator=MIMO_C(5,5).den{1}
  R3 Controller : DiscreteTransferFcn  Numerator=MIMO_C(6,6).num{1}  Denominator=MIMO_C(6,6).den{1}
  T1 Controller : DiscreteTransferFcn  Numerator=MIMO_C(1,1).num{1}  Denominator=MIMO_C(1,1).den{1}
  T2 Controller : DiscreteTransferFcn  Numerator=MIMO_C(2,2).num{1}  Denominator=MIMO_C(2,2).den{1}
  T3 Controller : DiscreteTransferFcn  Numerator=MIMO_C(3,3).num{1}  Denominator=MIMO_C(3,3).den{1}
  Out1 : Outport
  wires:
  In1/1 -> Demux1/1
  Demux1/1 -> Gain/1
  Demux1/2 -> Gain1/1
  Demux1/3 -> Gain5/1
  Demux1/4 -> Gain2/1
  Demux1/5 -> Gain3/1
  Demux1/6 -> Gain4/1
  R3 Controller/1 -> Mux1/6
  R2 Controller/1 -> Mux1/5
  R1 Controller/1 -> Mux1/4
  T3 Controller/1 -> Mux1/3
  T2 Controller/1 -> Mux1/2
  T1 Controller/1 -> Mux1/1
  Mux1/1 -> Out1/1
  Gain/1 -> T1 Controller/1
  Gain1/1 -> T2 Controller/1
  Gain2/1 -> R1 Controller/1
  Gain3/1 -> R2 Controller/1
  Gain4/1 -> R3 Controller/1
  Gain5/1 -> T3 Controller/1

== system AcO_Ctrl_Geometric_headless_R2016a/Structural Dynamics V3.3/Structural Dynamics V3.3a/Structural Dynamics Plus CL Az El M1 force/M1 Force Control/ControlM1S4/MIMO Controller ==
  In1 : Inport
  Demux1 : Demux  Outputs=6
  Gain{,1..5} (6 alike) : Gain
  Mux1 : Mux  Inputs=6
  R1 Controller : DiscreteTransferFcn  Numerator=MIMO_C(4,4).num{1}  Denominator=MIMO_C(4,4).den{1}
  R2 Controller : DiscreteTransferFcn  Numerator=MIMO_C(5,5).num{1}  Denominator=MIMO_C(5,5).den{1}
  R3 Controller : DiscreteTransferFcn  Numerator=MIMO_C(6,6).num{1}  Denominator=MIMO_C(6,6).den{1}
  T1 Controller : DiscreteTransferFcn  Numerator=MIMO_C(1,1).num{1}  Denominator=MIMO_C(1,1).den{1}
  T2 Controller : DiscreteTransferFcn  Numerator=MIMO_C(2,2).num{1}  Denominator=MIMO_C(2,2).den{1}
  T3 Controller : DiscreteTransferFcn  Numerator=MIMO_C(3,3).num{1}  Denominator=MIMO_C(3,3).den{1}
  Out1 : Outport
  wires:
  Gain5/1 -> T3 Controller/1
  Gain4/1 -> R3 Controller/1
  Gain3/1 -> R2 Controller/1
  Gain2/1 -> R1 Controller/1
  Gain1/1 -> T2 Controller/1
  Gain/1 -> T1 Controller/1
  Mux1/1 -> Out1/1
  T1 Controller/1 -> Mux1/1
  T2 Controller/1 -> Mux1/2
  T3 Controller/1 -> Mux1/3
  R1 Controller/1 -> Mux1/4
  R2 Controller/1 -> Mux1/5
  R3 Controller/1 -> Mux1/6
  Demux1/6 -> Gain4/1
  Demux1/5 -> Gain3/1
  Demux1/4 -> Gain2/1
  Demux1/3 -> Gain5/1
  Demux1/2 -> Gain1/1
  Demux1/1 -> Gain/1
  In1/1 -> Demux1/1

== system AcO_Ctrl_Geometric_headless_R2016a/Structural Dynamics V3.3/Structural Dynamics V3.3a/Structural Dynamics Plus CL Az El M1 force/M1 Force Control/ControlM1S5/MIMO Controller ==
  In1 : Inport
  Demux1 : Demux  Outputs=6
  Gain{,1..5} (6 alike) : Gain
  Mux1 : Mux  Inputs=6
  R1 Controller : DiscreteTransferFcn  Numerator=MIMO_C(4,4).num{1}  Denominator=MIMO_C(4,4).den{1}
  R2 Controller : DiscreteTransferFcn  Numerator=MIMO_C(5,5).num{1}  Denominator=MIMO_C(5,5).den{1}
  R3 Controller : DiscreteTransferFcn  Numerator=MIMO_C(6,6).num{1}  Denominator=MIMO_C(6,6).den{1}
  T1 Controller : DiscreteTransferFcn  Numerator=MIMO_C(1,1).num{1}  Denominator=MIMO_C(1,1).den{1}
  T2 Controller : DiscreteTransferFcn  Numerator=MIMO_C(2,2).num{1}  Denominator=MIMO_C(2,2).den{1}
  T3 Controller : DiscreteTransferFcn  Numerator=MIMO_C(3,3).num{1}  Denominator=MIMO_C(3,3).den{1}
  Out1 : Outport
  wires:
  In1/1 -> Demux1/1
  Demux1/1 -> Gain/1
  Demux1/2 -> Gain1/1
  Demux1/3 -> Gain5/1
  Demux1/4 -> Gain2/1
  Demux1/5 -> Gain3/1
  Demux1/6 -> Gain4/1
  R3 Controller/1 -> Mux1/6
  R2 Controller/1 -> Mux1/5
  R1 Controller/1 -> Mux1/4
  T3 Controller/1 -> Mux1/3
  T2 Controller/1 -> Mux1/2
  T1 Controller/1 -> Mux1/1
  Mux1/1 -> Out1/1
  Gain/1 -> T1 Controller/1
  Gain1/1 -> T2 Controller/1
  Gain2/1 -> R1 Controller/1
  Gain3/1 -> R2 Controller/1
  Gain4/1 -> R3 Controller/1
  Gain5/1 -> T3 Controller/1

== system AcO_Ctrl_Geometric_headless_R2016a/Structural Dynamics V3.3/Structural Dynamics V3.3a/Structural Dynamics Plus CL Az El M1 force/M1 Force Control/ControlM1S6/MIMO Controller ==
  In1 : Inport
  Demux1 : Demux  Outputs=6
  Gain{,1..5} (6 alike) : Gain
  Mux1 : Mux  Inputs=6
  R1 Controller : DiscreteTransferFcn  Numerator=MIMO_C(4,4).num{1}  Denominator=MIMO_C(4,4).den{1}
  R2 Controller : DiscreteTransferFcn  Numerator=MIMO_C(5,5).num{1}  Denominator=MIMO_C(5,5).den{1}
  R3 Controller : DiscreteTransferFcn  Numerator=MIMO_C(6,6).num{1}  Denominator=MIMO_C(6,6).den{1}
  T1 Controller : DiscreteTransferFcn  Numerator=MIMO_C(1,1).num{1}  Denominator=MIMO_C(1,1).den{1}
  T2 Controller : DiscreteTransferFcn  Numerator=MIMO_C(2,2).num{1}  Denominator=MIMO_C(2,2).den{1}
  T3 Controller : DiscreteTransferFcn  Numerator=MIMO_C(3,3).num{1}  Denominator=MIMO_C(3,3).den{1}
  Out1 : Outport
  wires:
  Gain5/1 -> T3 Controller/1
  Gain4/1 -> R3 Controller/1
  Gain3/1 -> R2 Controller/1
  Gain2/1 -> R1 Controller/1
  Gain1/1 -> T2 Controller/1
  Gain/1 -> T1 Controller/1
  Mux1/1 -> Out1/1
  T1 Controller/1 -> Mux1/1
  T2 Controller/1 -> Mux1/2
  T3 Controller/1 -> Mux1/3
  R1 Controller/1 -> Mux1/4
  R2 Controller/1 -> Mux1/5
  R3 Controller/1 -> Mux1/6
  Demux1/6 -> Gain4/1
  Demux1/5 -> Gain3/1
  Demux1/4 -> Gain2/1
  Demux1/3 -> Gain5/1
  Demux1/2 -> Gain1/1
  Demux1/1 -> Gain/1
  In1/1 -> Demux1/1

== system AcO_Ctrl_Geometric_headless_R2016a/Structural Dynamics V3.3/Structural Dynamics V3.3a/Structural Dynamics Plus CL Az El M1 force/M1 Force Control/ControlM1S7/MIMO Controller ==
  In1 : Inport
  Demux1 : Demux  Outputs=6
  Gain{,1..5} (6 alike) : Gain
  Mux1 : Mux  Inputs=6
  R1 Controller : DiscreteTransferFcn  Numerator=MIMO_C(4,4).num{1}  Denominator=MIMO_C(4,4).den{1}
  R2 Controller : DiscreteTransferFcn  Numerator=MIMO_C(5,5).num{1}  Denominator=MIMO_C(5,5).den{1}
  R3 Controller : DiscreteTransferFcn  Numerator=MIMO_C(6,6).num{1}  Denominator=MIMO_C(6,6).den{1}
  T1 Controller : DiscreteTransferFcn  Numerator=MIMO_C(1,1).num{1}  Denominator=MIMO_C(1,1).den{1}
  T2 Controller : DiscreteTransferFcn  Numerator=MIMO_C(2,2).num{1}  Denominator=MIMO_C(2,2).den{1}
  T3 Controller : DiscreteTransferFcn  Numerator=MIMO_C(3,3).num{1}  Denominator=MIMO_C(3,3).den{1}
  Out1 : Outport
  wires:
  Gain5/1 -> T3 Controller/1
  Gain4/1 -> R3 Controller/1
  Gain3/1 -> R2 Controller/1
  Gain2/1 -> R1 Controller/1
  Gain1/1 -> T2 Controller/1
  Gain/1 -> T1 Controller/1
  Mux1/1 -> Out1/1
  T1 Controller/1 -> Mux1/1
  T2 Controller/1 -> Mux1/2
  T3 Controller/1 -> Mux1/3
  R1 Controller/1 -> Mux1/4
  R2 Controller/1 -> Mux1/5
  R3 Controller/1 -> Mux1/6
  Demux1/6 -> Gain4/1
  Demux1/5 -> Gain3/1
  Demux1/4 -> Gain2/1
  Demux1/3 -> Gain5/1
  Demux1/2 -> Gain1/1
  Demux1/1 -> Gain/1
  In1/1 -> Demux1/1

== system AcO_Ctrl_Geometric_headless_R2016a/Structural Dynamics V3.3/Structural Dynamics V3.5.2/Structural Dynamics Plus CL Az El M1 force/M1 Force Control/ControlM1S1/MIMO Controller ==
  In1 : Inport
  Demux1 : Demux  Outputs=6
  Gain{,1..5} (6 alike) : Gain
  Mux1 : Mux  Inputs=6
  R1 Controller : DiscreteTransferFcn  Numerator=MIMO_C(4,4).num{1}  Denominator=MIMO_C(4,4).den{1}
  R2 Controller : DiscreteTransferFcn  Numerator=MIMO_C(5,5).num{1}  Denominator=MIMO_C(5,5).den{1}
  R3 Controller : DiscreteTransferFcn  Numerator=MIMO_C(6,6).num{1}  Denominator=MIMO_C(6,6).den{1}
  T1 Controller : DiscreteTransferFcn  Numerator=MIMO_C(1,1).num{1}  Denominator=MIMO_C(1,1).den{1}
  T2 Controller : DiscreteTransferFcn  Numerator=MIMO_C(2,2).num{1}  Denominator=MIMO_C(2,2).den{1}
  T3 Controller : DiscreteTransferFcn  Numerator=MIMO_C(3,3).num{1}  Denominator=MIMO_C(3,3).den{1}
  Out1 : Outport
  wires:
  Gain5/1 -> T3 Controller/1
  Gain4/1 -> R3 Controller/1
  Gain3/1 -> R2 Controller/1
  Gain2/1 -> R1 Controller/1
  Gain1/1 -> T2 Controller/1
  Gain/1 -> T1 Controller/1
  Mux1/1 -> Out1/1
  T1 Controller/1 -> Mux1/1
  T2 Controller/1 -> Mux1/2
  T3 Controller/1 -> Mux1/3
  R1 Controller/1 -> Mux1/4
  R2 Controller/1 -> Mux1/5
  R3 Controller/1 -> Mux1/6
  Demux1/6 -> Gain4/1
  Demux1/5 -> Gain3/1
  Demux1/4 -> Gain2/1
  Demux1/3 -> Gain5/1
  Demux1/2 -> Gain1/1
  Demux1/1 -> Gain/1
  In1/1 -> Demux1/1

== system AcO_Ctrl_Geometric_headless_R2016a/Structural Dynamics V3.3/Structural Dynamics V3.5.2/Structural Dynamics Plus CL Az El M1 force/M1 Force Control/ControlM1S2/MIMO Controller ==
  In1 : Inport
  Demux1 : Demux  Outputs=6
  Gain{,1..5} (6 alike) : Gain
  Mux1 : Mux  Inputs=6
  R1 Controller : DiscreteTransferFcn  Numerator=MIMO_C(4,4).num{1}  Denominator=MIMO_C(4,4).den{1}
  R2 Controller : DiscreteTransferFcn  Numerator=MIMO_C(5,5).num{1}  Denominator=MIMO_C(5,5).den{1}
  R3 Controller : DiscreteTransferFcn  Numerator=MIMO_C(6,6).num{1}  Denominator=MIMO_C(6,6).den{1}
  T1 Controller : DiscreteTransferFcn  Numerator=MIMO_C(1,1).num{1}  Denominator=MIMO_C(1,1).den{1}
  T2 Controller : DiscreteTransferFcn  Numerator=MIMO_C(2,2).num{1}  Denominator=MIMO_C(2,2).den{1}
  T3 Controller : DiscreteTransferFcn  Numerator=MIMO_C(3,3).num{1}  Denominator=MIMO_C(3,3).den{1}
  Out1 : Outport
  wires:
  In1/1 -> Demux1/1
  Demux1/1 -> Gain/1
  Demux1/2 -> Gain1/1
  Demux1/3 -> Gain5/1
  Demux1/4 -> Gain2/1
  Demux1/5 -> Gain3/1
  Demux1/6 -> Gain4/1
  R3 Controller/1 -> Mux1/6
  R2 Controller/1 -> Mux1/5
  R1 Controller/1 -> Mux1/4
  T3 Controller/1 -> Mux1/3
  T2 Controller/1 -> Mux1/2
  T1 Controller/1 -> Mux1/1
  Mux1/1 -> Out1/1
  Gain/1 -> T1 Controller/1
  Gain1/1 -> T2 Controller/1
  Gain2/1 -> R1 Controller/1
  Gain3/1 -> R2 Controller/1
  Gain4/1 -> R3 Controller/1
  Gain5/1 -> T3 Controller/1

== system AcO_Ctrl_Geometric_headless_R2016a/Structural Dynamics V3.3/Structural Dynamics V3.5.2/Structural Dynamics Plus CL Az El M1 force/M1 Force Control/ControlM1S3/MIMO Controller ==
  In1 : Inport
  Demux1 : Demux  Outputs=6
  Gain{,1..5} (6 alike) : Gain
  Mux1 : Mux  Inputs=6
  R1 Controller : DiscreteTransferFcn  Numerator=MIMO_C(4,4).num{1}  Denominator=MIMO_C(4,4).den{1}
  R2 Controller : DiscreteTransferFcn  Numerator=MIMO_C(5,5).num{1}  Denominator=MIMO_C(5,5).den{1}
  R3 Controller : DiscreteTransferFcn  Numerator=MIMO_C(6,6).num{1}  Denominator=MIMO_C(6,6).den{1}
  T1 Controller : DiscreteTransferFcn  Numerator=MIMO_C(1,1).num{1}  Denominator=MIMO_C(1,1).den{1}
  T2 Controller : DiscreteTransferFcn  Numerator=MIMO_C(2,2).num{1}  Denominator=MIMO_C(2,2).den{1}
  T3 Controller : DiscreteTransferFcn  Numerator=MIMO_C(3,3).num{1}  Denominator=MIMO_C(3,3).den{1}
  Out1 : Outport
  wires:
  Gain5/1 -> T3 Controller/1
  Gain4/1 -> R3 Controller/1
  Gain3/1 -> R2 Controller/1
  Gain2/1 -> R1 Controller/1
  Gain1/1 -> T2 Controller/1
  Gain/1 -> T1 Controller/1
  Mux1/1 -> Out1/1
  T1 Controller/1 -> Mux1/1
  T2 Controller/1 -> Mux1/2
  T3 Controller/1 -> Mux1/3
  R1 Controller/1 -> Mux1/4
  R2 Controller/1 -> Mux1/5
  R3 Controller/1 -> Mux1/6
  Demux1/6 -> Gain4/1
  Demux1/5 -> Gain3/1
  Demux1/4 -> Gain2/1
  Demux1/3 -> Gain5/1
  Demux1/2 -> Gain1/1
  Demux1/1 -> Gain/1
  In1/1 -> Demux1/1

== system AcO_Ctrl_Geometric_headless_R2016a/Structural Dynamics V3.3/Structural Dynamics V3.5.2/Structural Dynamics Plus CL Az El M1 force/M1 Force Control/ControlM1S4/MIMO Controller ==
  In1 : Inport
  Demux1 : Demux  Outputs=6
  Gain{,1..5} (6 alike) : Gain
  Mux1 : Mux  Inputs=6
  R1 Controller : DiscreteTransferFcn  Numerator=MIMO_C(4,4).num{1}  Denominator=MIMO_C(4,4).den{1}
  R2 Controller : DiscreteTransferFcn  Numerator=MIMO_C(5,5).num{1}  Denominator=MIMO_C(5,5).den{1}
  R3 Controller : DiscreteTransferFcn  Numerator=MIMO_C(6,6).num{1}  Denominator=MIMO_C(6,6).den{1}
  T1 Controller : DiscreteTransferFcn  Numerator=MIMO_C(1,1).num{1}  Denominator=MIMO_C(1,1).den{1}
  T2 Controller : DiscreteTransferFcn  Numerator=MIMO_C(2,2).num{1}  Denominator=MIMO_C(2,2).den{1}
  T3 Controller : DiscreteTransferFcn  Numerator=MIMO_C(3,3).num{1}  Denominator=MIMO_C(3,3).den{1}
  Out1 : Outport
  wires:
  In1/1 -> Demux1/1
  Demux1/1 -> Gain/1
  Demux1/2 -> Gain1/1
  Demux1/3 -> Gain5/1
  Demux1/4 -> Gain2/1
  Demux1/5 -> Gain3/1
  Demux1/6 -> Gain4/1
  R3 Controller/1 -> Mux1/6
  R2 Controller/1 -> Mux1/5
  R1 Controller/1 -> Mux1/4
  T3 Controller/1 -> Mux1/3
  T2 Controller/1 -> Mux1/2
  T1 Controller/1 -> Mux1/1
  Mux1/1 -> Out1/1
  Gain/1 -> T1 Controller/1
  Gain1/1 -> T2 Controller/1
  Gain2/1 -> R1 Controller/1
  Gain3/1 -> R2 Controller/1
  Gain4/1 -> R3 Controller/1
  Gain5/1 -> T3 Controller/1

== system AcO_Ctrl_Geometric_headless_R2016a/Structural Dynamics V3.3/Structural Dynamics V3.5.2/Structural Dynamics Plus CL Az El M1 force/M1 Force Control/ControlM1S5/MIMO Controller ==
  In1 : Inport
  Demux1 : Demux  Outputs=6
  Gain{,1..5} (6 alike) : Gain
  Mux1 : Mux  Inputs=6
  R1 Controller : DiscreteTransferFcn  Numerator=MIMO_C(4,4).num{1}  Denominator=MIMO_C(4,4).den{1}
  R2 Controller : DiscreteTransferFcn  Numerator=MIMO_C(5,5).num{1}  Denominator=MIMO_C(5,5).den{1}
  R3 Controller : DiscreteTransferFcn  Numerator=MIMO_C(6,6).num{1}  Denominator=MIMO_C(6,6).den{1}
  T1 Controller : DiscreteTransferFcn  Numerator=MIMO_C(1,1).num{1}  Denominator=MIMO_C(1,1).den{1}
  T2 Controller : DiscreteTransferFcn  Numerator=MIMO_C(2,2).num{1}  Denominator=MIMO_C(2,2).den{1}
  T3 Controller : DiscreteTransferFcn  Numerator=MIMO_C(3,3).num{1}  Denominator=MIMO_C(3,3).den{1}
  Out1 : Outport
  wires:
  Gain5/1 -> T3 Controller/1
  Gain4/1 -> R3 Controller/1
  Gain3/1 -> R2 Controller/1
  Gain2/1 -> R1 Controller/1
  Gain1/1 -> T2 Controller/1
  Gain/1 -> T1 Controller/1
  Mux1/1 -> Out1/1
  T1 Controller/1 -> Mux1/1
  T2 Controller/1 -> Mux1/2
  T3 Controller/1 -> Mux1/3
  R1 Controller/1 -> Mux1/4
  R2 Controller/1 -> Mux1/5
  R3 Controller/1 -> Mux1/6
  Demux1/6 -> Gain4/1
  Demux1/5 -> Gain3/1
  Demux1/4 -> Gain2/1
  Demux1/3 -> Gain5/1
  Demux1/2 -> Gain1/1
  Demux1/1 -> Gain/1
  In1/1 -> Demux1/1

== system AcO_Ctrl_Geometric_headless_R2016a/Structural Dynamics V3.3/Structural Dynamics V3.5.2/Structural Dynamics Plus CL Az El M1 force/M1 Force Control/ControlM1S6/MIMO Controller ==
  In1 : Inport
  Demux1 : Demux  Outputs=6
  Gain{,1..5} (6 alike) : Gain
  Mux1 : Mux  Inputs=6
  R1 Controller : DiscreteTransferFcn  Numerator=MIMO_C(4,4).num{1}  Denominator=MIMO_C(4,4).den{1}
  R2 Controller : DiscreteTransferFcn  Numerator=MIMO_C(5,5).num{1}  Denominator=MIMO_C(5,5).den{1}
  R3 Controller : DiscreteTransferFcn  Numerator=MIMO_C(6,6).num{1}  Denominator=MIMO_C(6,6).den{1}
  T1 Controller : DiscreteTransferFcn  Numerator=MIMO_C(1,1).num{1}  Denominator=MIMO_C(1,1).den{1}
  T2 Controller : DiscreteTransferFcn  Numerator=MIMO_C(2,2).num{1}  Denominator=MIMO_C(2,2).den{1}
  T3 Controller : DiscreteTransferFcn  Numerator=MIMO_C(3,3).num{1}  Denominator=MIMO_C(3,3).den{1}
  Out1 : Outport
  wires:
  In1/1 -> Demux1/1
  Demux1/1 -> Gain/1
  Demux1/2 -> Gain1/1
  Demux1/3 -> Gain5/1
  Demux1/4 -> Gain2/1
  Demux1/5 -> Gain3/1
  Demux1/6 -> Gain4/1
  R3 Controller/1 -> Mux1/6
  R2 Controller/1 -> Mux1/5
  R1 Controller/1 -> Mux1/4
  T3 Controller/1 -> Mux1/3
  T2 Controller/1 -> Mux1/2
  T1 Controller/1 -> Mux1/1
  Mux1/1 -> Out1/1
  Gain/1 -> T1 Controller/1
  Gain1/1 -> T2 Controller/1
  Gain2/1 -> R1 Controller/1
  Gain3/1 -> R2 Controller/1
  Gain4/1 -> R3 Controller/1
  Gain5/1 -> T3 Controller/1

== system AcO_Ctrl_Geometric_headless_R2016a/Structural Dynamics V3.3/Structural Dynamics V3.5.2/Structural Dynamics Plus CL Az El M1 force/M1 Force Control/ControlM1S7/MIMO Controller ==
  In1 : Inport
  Demux1 : Demux  Outputs=6
  Gain{,1..5} (6 alike) : Gain
  Mux1 : Mux  Inputs=6
  R1 Controller : DiscreteTransferFcn  Numerator=MIMO_C(4,4).num{1}  Denominator=MIMO_C(4,4).den{1}
  R2 Controller : DiscreteTransferFcn  Numerator=MIMO_C(5,5).num{1}  Denominator=MIMO_C(5,5).den{1}
  R3 Controller : DiscreteTransferFcn  Numerator=MIMO_C(6,6).num{1}  Denominator=MIMO_C(6,6).den{1}
  T1 Controller : DiscreteTransferFcn  Numerator=MIMO_C(1,1).num{1}  Denominator=MIMO_C(1,1).den{1}
  T2 Controller : DiscreteTransferFcn  Numerator=MIMO_C(2,2).num{1}  Denominator=MIMO_C(2,2).den{1}
  T3 Controller : DiscreteTransferFcn  Numerator=MIMO_C(3,3).num{1}  Denominator=MIMO_C(3,3).den{1}
  Out1 : Outport
  wires:
  Gain5/1 -> T3 Controller/1
  Gain4/1 -> R3 Controller/1
  Gain3/1 -> R2 Controller/1
  Gain2/1 -> R1 Controller/1
  Gain1/1 -> T2 Controller/1
  Gain/1 -> T1 Controller/1
  Mux1/1 -> Out1/1
  T1 Controller/1 -> Mux1/1
  T2 Controller/1 -> Mux1/2
  T3 Controller/1 -> Mux1/3
  R1 Controller/1 -> Mux1/4
  R2 Controller/1 -> Mux1/5
  R3 Controller/1 -> Mux1/6
  Demux1/6 -> Gain4/1
  Demux1/5 -> Gain3/1
  Demux1/4 -> Gain2/1
  Demux1/3 -> Gain5/1
  Demux1/2 -> Gain1/1
  Demux1/1 -> Gain/1
  In1/1 -> Demux1/1
